simulink subsystem "mission_manager_interface_cgn"  (R2025b)
settings: Solver=VariableStepAuto  StartTime=0.0  StopTime=10.0  RelTol=1e-3
undefined symbols (not defined in the file or in its folder): dt_control
libraries: ros2lib x2
settings Model: Creator=vulcangrip  LastModifiedBy=vulcangrip

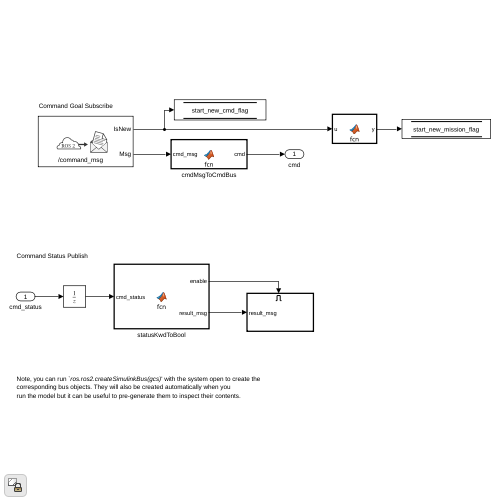
[thumbnail: Simulink's stored preview of the top-level diagram]
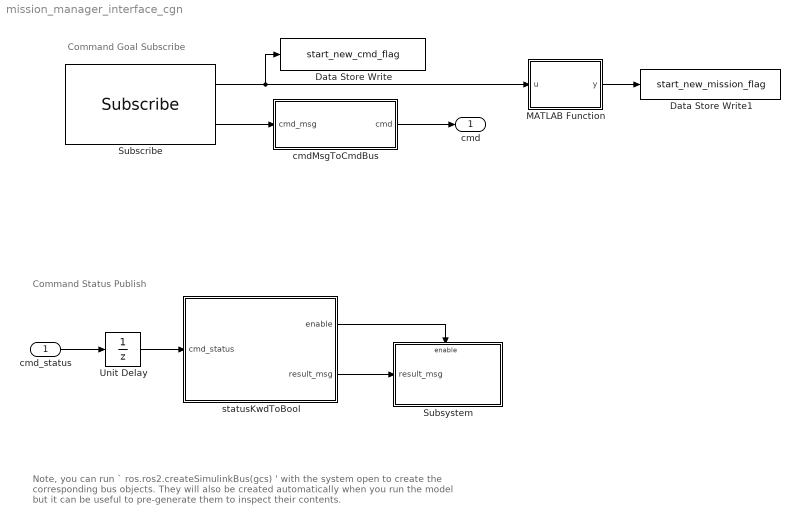
== system mission_manager_interface_cgn ==
  note: Command Goal Subscribe
  note: Note, you can run ` ros.ros2.createSimulinkBus(gcs) ' with the system open to create the
      | corresponding bus objects. They will also be created automatically when you
      | run the model but it can be useful to pre-generate them to inspect their contents.
  note: Command Status Publish
  cmd_status : Inport  SampleTime=dt_control
  Data Store Write : DataStoreWrite  DataStoreName=start_new_cmd_flag  IndexOptions=Index vector (dialog)  Indices=1  OutputSizes=1
  Data Store Write1 : DataStoreWrite  DataStoreName=start_new_mission_flag  IndexOptions=Index vector (dialog)  Indices=1  OutputSizes=1
  MATLAB Function : MATLAB Function  TreatAsAtomicUnit=on
  Subscribe : ros2lib/Subscribe  topicSource=Specify your own  topic=/command_msg  messageType=custom_interfaces/Goal  sampleTime=0.01  QOSHistory=Keep last  QOSDepth=10  QOSReliability=Reliable  QOSDurability=Volatile  QOSDeadline=Inf  QOSLifespan=Inf  QOSLiveliness=Automatic  QOSLeaseDuration=Inf  QOSAvoidROSNamespaceConventions=off
  Subsystem : Subsystem
  Unit Delay : UnitDelay  SampleTime=-1  HasFrameUpgradeWarning=on
  cmdMsgToCmdBus : MATLAB Function  TreatAsAtomicUnit=on
  statusKwdToBool : MATLAB Function  TreatAsAtomicUnit=on
  cmd : Outport  SampleTime=dt_control
  wires:
  cmdMsgToCmdBus/1(cmd) -> cmd/1
  Subscribe/2 -> cmdMsgToCmdBus/1(cmd_msg)
  statusKwdToBool/1(enable) -> Subsystem/Enable
  statusKwdToBool/2(result_msg) -> Subsystem/1(result_msg)
  Subscribe/1 -> MATLAB Function/1(u), Data Store Write/1
  cmd_status/1 -> Unit Delay/1
  Unit Delay/1 -> statusKwdToBool/1(cmd_status)
  MATLAB Function/1(y) -> Data Store Write1/1

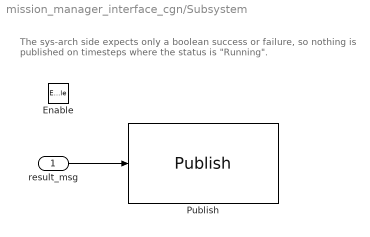
== system mission_manager_interface_cgn/Subsystem ==
  note: The sys-arch side expects only a boolean success or failure, so nothing
      | is published on timesteps where the status is "Running".
  result_msg : Inport
  Enable : EnablePort
  Publish : ros2lib/Publish  topicSource=Specify your own  topic=/command_result  messageType=custom_interfaces/Result  QOSHistory=Keep last  QOSDepth=10  QOSReliability=Reliable  QOSDurability=Volatile  QOSDeadline=Inf  QOSLifespan=Inf  QOSLiveliness=Automatic  QOSLeaseDuration=Inf  QOSAvoidROSNamespaceConventions=off
  wires:
  result_msg/1 -> Publish/1

== matlab function mission_manager_interface_cgn/MATLAB Function ==
  data: u input; y output
function y = fcn(u)
persistent start_new_mission_flag

if isempty(start_new_mission_flag)
    start_new_mission_flag = true;
end

if(u)
    start_new_mission_flag = false;
end

y = start_new_mission_flag;

== matlab function mission_manager_interface_cgn/cmdMsgToCmdBus ==
  data: cmd_msg input Bus: SL_Bus_custom_interfaces_Goal; cmd output Bus: cmd_bus
function cmd = fcn(cmd_msg)

cmd = cmdMsgToCmdBus(cmd_msg);

end

== matlab function mission_manager_interface_cgn/statusKwdToBool ==
  data: enable output; cmd_status input; result_msg output Bus: SL_Bus_custom_interfaces_Result
function [enable, result_msg]   = fcn(cmd_status)

[enable, result_msg] = statusKwdToBool(cmd_status);
